simulink model "s_ip02_position"  (Simulink 7.8)
settings: Solver=ode1  SolverMode=SingleTasking  StartTime=0.0  StopTime=5  FixedStep=0.001  RelTol=1e-3  AbsTol=1e-6
values from neighbouring files (symbols this model uses):
  K = Am / Beqv    [d_model_param.m]
  kp = wn^2/K*tau    [d_ip02_position.m]    (also in setup_ip02_position.m = 0)
  kv = (-1+2*zeta*wn*tau)/K    [d_ip02_position.m]    (also in setup_ip02_position.m = 0)
  tau = Jeq / Beqv    [d_model_param.m]
  wcf = 2 * pi * 50    (= 314.159265359)    [setup_ip02_position.m]
  zetaf = 0.9    [setup_ip02_position.m]
libraries: simulink x1
settings Model: Creator=MLevis  LastModifiedBy=pmartin  BufferReuse=off
settings DataIOCC: LimitDataPoints=off
settings OptimizationCC: BlockReduction=off  BooleanDataType=off  OptimizeBlockIOStorage=off  BufferReuse=off  ExpressionFolding=off  FoldNonRolledExpr=off  LocalBlockOutputs=off  InitFltsAndDblsToZero=on
settings DebuggingCC: SaveWithParameterizedLinksMsg=none  SignalResolutionControl=TryResolveAllWithWarning  SolverPrmCheckMsg=none  MultiTaskDSMMsg=warning  MultiTaskCondExecSysMsg=none  FcnCallInpInsideContextMsg=Use local settings  StrictBusMsg=None
settings HardwareCC: TargetUnknown=on
settings RTWCC: SystemTargetFile=wincon.tlc  MakeCommand=make_wc  TemplateMakefile=nt_msvc.tmf  ProcessScript=wincon_make_rtw_hook  IncludeERTFirstTime=on
settings STFCustomTargetCC: TargetFcnLib=ansi_tfl_tmw.mat  ModelReferenceCompliant=off  SystemTargetFile=wincon.tlc

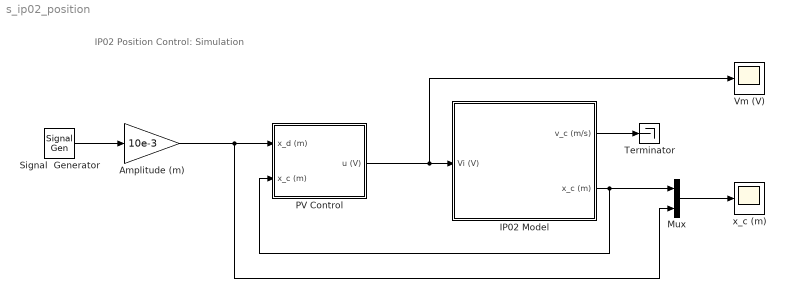
== system s_ip02_position ==
  note: IP02 Position Control: Simulation
  Amplitude (m) : Gain  Gain=10e-3  SaturateOnIntegerOverflow=on  OutDataTypeStr=Inherit: Same as input  ParamDataTypeStr=Inherit: Same as input
  IP02 Model : Subsystem
  Mux : Mux  Inputs=2
  PV Control : Subsystem
  Signal  Generator : SignalGenerator  WaveForm=square  Frequency=0.66
  Terminator : Terminator
  Vm (V) : Scope
      settings: SaveName=data_vm  DataFormat=Array
  x_c (m) : Scope
      settings: SaveName=data_pos  DataFormat=Array
  wires:
  Signal  Generator/1 -> Amplitude (m)/1
  Amplitude (m)/1 -> PV Control/1(x_d (m)), Mux/2
  PV Control/1(u (V)) -> IP02 Model/1(Vi (V)), Vm (V)/1
  IP02 Model/2(x_c (m)) -> PV Control/2(x_c (m)), Mux/1
  IP02 Model/1(v_c (m/s)) -> Terminator/1
  Mux/1 -> x_c (m)/1

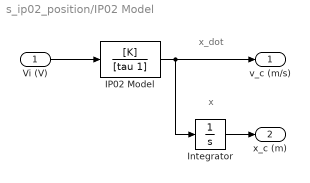
== system s_ip02_position/IP02 Model ==
  note: x_dot
  note: x
  Vi (V) : Inport
  IP02 Model : TransferFcn  Numerator=[K]  Denominator=[tau 1]
  Integrator : Integrator
  v_c (m/s) : Outport
  x_c (m) : Outport  Port=2
  wires:
  IP02 Model/1 -> v_c (m/s)/1, Integrator/1
  Vi (V)/1 -> IP02 Model/1
  Integrator/1 -> x_c (m)/1

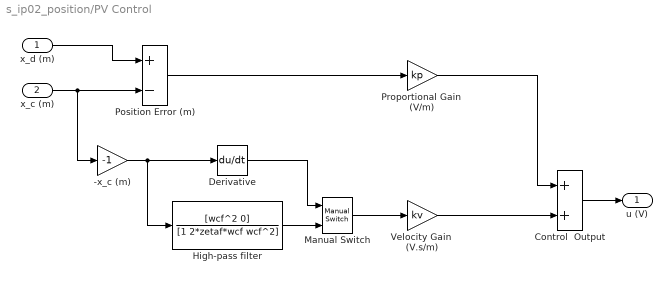
== system s_ip02_position/PV Control ==
  x_d (m) : Inport
  x_c (m) : Inport  Port=2
  -x_c (m) : Gain  Gain=-1
  Control  Output : Sum
  Derivative : Derivative
  High-pass filter : TransferFcn  Numerator=[wcf^2 0]  Denominator=[1 2*zetaf*wcf wcf^2]
  Manual Switch : simulink/Signal Routing/Manual Switch  sw=0  action=0  varsize=off
  Position Error (m) : Sum  Inputs=+-
  Proportional Gain  (V/m) : Gain  Gain=kp
  Velocity Gain  (V.s/m) : Gain  Gain=kv
  u (V) : Outport
  wires:
  Proportional Gain  (V/m)/1 -> Control  Output/1
  x_d (m)/1 -> Position Error (m)/1
  Control  Output/1 -> u (V)/1
  x_c (m)/1 -> Position Error (m)/2, -x_c (m)/1
  Position Error (m)/1 -> Proportional Gain  (V/m)/1
  -x_c (m)/1 -> Derivative/1, High-pass filter/1
  High-pass filter/1 -> Manual Switch/2
  Manual Switch/1 -> Velocity Gain  (V.s/m)/1
  Derivative/1 -> Manual Switch/1
  Velocity Gain  (V.s/m)/1 -> Control  Output/2
